simulink model "task_2_0"  (R2023a)
settings: Solver=VariableStepAuto  StartTime=0.0  StopTime=50.0  RelTol=1e-8
model workspace (MAT data in the model file):
  T1 = Simulink.Parameter
  T1.DataType = 'auto'
  T1.Complexity = 'real'
  T1.Dimensions = [0 0]
  T2 = Simulink.Parameter
  T2.DataType = 'auto'
  T2.Complexity = 'real'
  T2.Dimensions = [0 0]
settings Model: Creator=user  LastModifiedBy=user

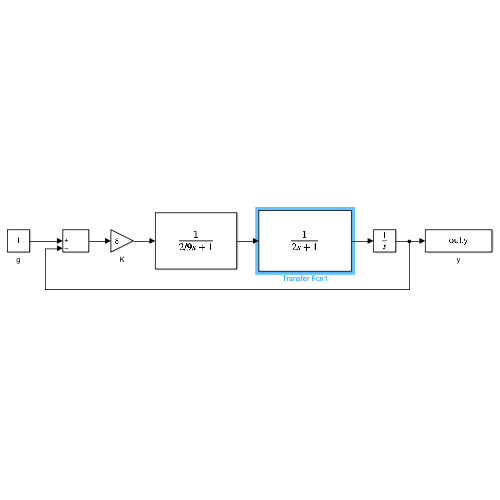
[thumbnail: Simulink's stored preview of the top-level diagram]
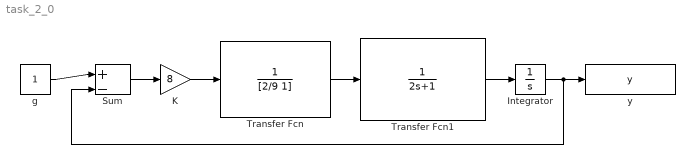
== system task_2_0 ==
  Integrator : Integrator
  K : Gain  Gain=8
  Sum : Sum  Inputs=|+-
  Transfer Fcn : TransferFcn  Denominator=[2/9 1]
  Transfer Fcn1 : TransferFcn  Denominator=[2 1]
  g : Constant
  y : ToWorkspace  VariableName=y  SaveFormat=Timeseries  SampleTime=-1
  wires:
  Transfer Fcn/1 -> Transfer Fcn1/1
  Integrator/1 -> Sum/2, y/1
  Sum/1 -> K/1
  K/1 -> Transfer Fcn/1
  Transfer Fcn1/1 -> Integrator/1
  g/1 -> Sum/1
